simulink model "master_thesis_simulink"  (R2022a)
settings: Solver=VariableStepAuto  StartTime=0.0  StopTime=p_0p.time(end)  FixedStep=0.001  RelTol=1e-3
values from neighbouring files (symbols this model uses):
  markers_forearm = [0.00210510253906 -0.143263397217 -0.00798474121094]    [markers_forearm.mat]
  markers_shoulder = [0.010127746582 -0.151647644043 -0.0119686279297]    [markers_shoulder.mat]
undefined symbols (not defined in the file or in its folder): arm, DiscIntNeverNeededParam, Discrete, ekf, kf, LS, m, markers_hand, n, noise, q0, q0_LS, q0_model, sample_Time, selected, state_observer, Time, tSh_0_0Conf, X, Y, Z
libraries: sm_lib x2029, nesl_utility x1553, robotlib x75, ctrlSharedLib x8
(part 6 of 70)

== system master_thesis_simulink/Experiments/S1_F1_H2/Human arm1/RightHand ==
  B_wrist__setting : sm_lib/Frames and Transforms/Rigid Transform  TranslationMethod=Cartesian  TranslationStandardOffset=0  TranslationLengthUnit=m  TranslationStandardAxis=+Z  TranslationCartesianOffset=[0, arm.hand.dimensions(2)/2, 0]  TranslationROffset=0  TranslationROffsetUnits=m  TranslationZOffset=0  TranslationZOffsetUnits=m  TranslationThetaOffset=0  TranslationThetaOffsetUnits=deg  RotationMethod=None  RotationAngleUnits=deg  RotationStandardAxis=+Z  RotationAngle=0.0  RotationArbitraryAxis=[0 0 1]  FollAlignAxisA=+X  BaseAlignAxisA=+Y  FollAlignAxisB=+Y  BaseAlignAxisB=+Z  RotationSequenceAxes=BaseAxes  RotationSequence=XYZ  RotationSequenceAngles=[0, 0, 0]  RotationSequenceAnglesUnits=rad  RotationMatrix=[1 0 0; 0 1 0; 0 0 1]
  Hand : sm_lib/Body Elements/Brick Solid  GraphicAmbientColor=[0.15 0.15 0.15 1.0]  BasedOnType=Density  BrickDimensions=arm.hand.dimensions  BrickDimensionUnits=m  CenterOfMass=[0, 0, 0]  CenterOfMassUnits=m  GraphicDiffuseColor=[1.0 0.6 0.4]  Density=1000  DensityUnits=kg/m^3  DoExposeReferenceFrame=on  GraphicEmissiveColor=[0.0 0.0 0.0 1.0]  ExportEntireGeometry=off  SerializedFrames=<Frames/>  MarkerShape=Sphere  MarkerSize=10  GraphicType=FromGeometry  InertiaType=CalculateFromGeometry  Mass=0  MassUnits=kg  MomentsOfInertia=[0, 0, 0]  MomentsOfInertiaUnits=kg*m^2  GraphicOpacity=1  ProductsOfInertia=[0, 0, 0]  ProductsOfInertiaUnits=kg*m^2  GraphicShininess=75  GraphicSpecularColor=[0.5 0.5 0.5 1.0]  GraphicVisPropType=SimpleVisualProperties
  Inertia : sm_lib/Body Elements/Inertia  InertiaType=Custom  Mass=arm.hand.mass  MassUnits=kg  CenterOfMass=[0, 0, 0]  CenterOfMassUnits=m  MomentsOfInertia=arm.hand.moment_inertia  MomentsOfInertiaUnits=kg*m^2  ProductsOfInertia=[0, 0, 0]  ProductsOfInertiaUnits=kg*m^2  GraphicType=None  MarkerShape=Inertia  MarkerSize=20  GraphicVisPropType=SimpleVisualProperties  GraphicDiffuseColor=[0.5 0.5 0.5]  GraphicSpecularColor=[0.5 0.5 0.5 1.0]  GraphicAmbientColor=[0.15 0.15 0.15 1.0]  GraphicEmissiveColor=[0.0 0.0 0.0 1.0]  GraphicShininess=75  GraphicOpacity=1.0
  Mux : Mux  Inputs=3
  PS-Simulink Converter : nesl_utility/PS-Simulink Converter  PhysicalDomain=network_engine_domain  SubClassName=ps_output  LeftPortType=input  RightPortType=output  PseudoPeriodic=off  Frequencies=[]  VectorFormat=inherit  Unit=inherit  AffineConversion=off
      settings: SourceProductBaseCode=SS,PW,VE
  PS-Simulink Converter1 : nesl_utility/PS-Simulink Converter  PhysicalDomain=network_engine_domain  SubClassName=ps_output  LeftPortType=input  RightPortType=output  PseudoPeriodic=off  Frequencies=[]  VectorFormat=inherit  Unit=inherit  AffineConversion=off
      settings: SourceProductBaseCode=SS,PW,VE
  PS-Simulink Converter2 : nesl_utility/PS-Simulink Converter  PhysicalDomain=network_engine_domain  SubClassName=ps_output  LeftPortType=input  RightPortType=output  PseudoPeriodic=off  Frequencies=[]  VectorFormat=inherit  Unit=inherit  AffineConversion=off
      settings: SourceProductBaseCode=SS,PW,VE
  Reference Frame : sm_lib/Frames and Transforms/Reference Frame
  Scope : Scope
  Transform Sensor : sm_lib/Frames and Transforms/Transform Sensor  MeasurementFrame=World  SenseAngle=off  SenseAxis=off  SenseAngle1=off  SenseAngle2=off  SenseAngle3=off  SenseQ=off  SenseR=off  SenseOmegaX=off  SenseOmegaY=off  SenseOmegaZ=off  SenseOmega1=off  SenseOmega2=off  SenseOmega3=off  SenseQDot=off  SenseRDot=off  SenseAlphaX=off  SenseAlphaY=off  SenseAlphaZ=off  SenseAlpha1=off  SenseAlpha2=off  SenseAlpha3=off  SenseQDDot=off  SenseRDDot=off  SenseX=on  SenseY=on  SenseZ=on  SenseRad=off  SenseAzim=off  SenseDist=off  SenseInc=off  SenseXDot=off  SenseYDot=off  SenseZDot=off  SenseRadDot=off  SenseAzimDot=off  SenseDistDot=off  SenseIncDot=off  SenseXDDot=off  SenseYDDot=off  SenseZDDot=off  SenseRadDDot=off  SenseAzimDDot=off  SenseDistDDot=off  SenseIncDDot=off
  B_wrist : PMIOPort  Side=Left
  W : PMIOPort  Port=2  Side=Left
  wires:
  Mux/1 -> Scope/1
  PS-Simulink Converter/1 -> Mux/1  "wrist_posx"
  PS-Simulink Converter1/1 -> Mux/2  "wrist_posy"
  PS-Simulink Converter2/1 -> Mux/3  "wrist_posz"
  connections:
  B_wrist__setting/RConn1 -- Transform Sensor/RConn1 -- B_wrist/RConn1
  PS-Simulink Converter2/LConn1 -- Transform Sensor/RConn4
  PS-Simulink Converter/LConn1 -- Transform Sensor/RConn2
  PS-Simulink Converter1/LConn1 -- Transform Sensor/RConn3
  Transform Sensor/LConn1 -- W/RConn1
  B_wrist__setting/LConn1 -- Inertia/RConn1 -- Reference Frame/RConn1 -- Hand/RConn1

== system master_thesis_simulink/Experiments/S1_F1_H2/Human arm1/RightShoulder ==
  B_shoulder__F_shoulder : sm_lib/Frames and Transforms/Rigid Transform  TranslationMethod=Cartesian  TranslationStandardOffset=0  TranslationLengthUnit=m  TranslationStandardAxis=+Z  TranslationCartesianOffset=[0 -arm.shoulder.length 0]  TranslationROffset=0  TranslationROffsetUnits=m  TranslationZOffset=0  TranslationZOffsetUnits=m  TranslationThetaOffset=0  TranslationThetaOffsetUnits=deg  RotationMethod=None  RotationAngleUnits=deg  RotationStandardAxis=+Z  RotationAngle=0.0  RotationArbitraryAxis=[0 0 1]  FollAlignAxisA=+X  BaseAlignAxisA=+Y  FollAlignAxisB=+Y  BaseAlignAxisB=+Z  RotationSequenceAxes=FollowerAxes  RotationSequence=XYX  RotationSequenceAngles=[0 0 0]  RotationSequenceAnglesUnits=deg  RotationMatrix=[1 0 0; 0 1 0; 0 0 1]
  Inertia : sm_lib/Body Elements/Inertia  InertiaType=Custom  Mass=arm.shoulder.mass  MassUnits=kg  CenterOfMass=[0 0 0]  CenterOfMassUnits=m  MomentsOfInertia=arm.shoulder.moment_inertia  MomentsOfInertiaUnits=kg*m^2  ProductsOfInertia=[0 0 0]  ProductsOfInertiaUnits=kg*m^2  GraphicType=None  MarkerShape=Inertia  MarkerSize=20  GraphicVisPropType=SimpleVisualProperties  GraphicDiffuseColor=[0.5 0.5 0.5]  GraphicSpecularColor=[0.5 0.5 0.5 1.0]  GraphicAmbientColor=[0.15 0.15 0.15 1.0]  GraphicEmissiveColor=[0.0 0.0 0.0 1.0]  GraphicShininess=75  GraphicOpacity=1.0
  Mux : Mux  Inputs=3
  PS-Simulink Converter : nesl_utility/PS-Simulink Converter  PhysicalDomain=network_engine_domain  SubClassName=ps_output  LeftPortType=input  RightPortType=output  PseudoPeriodic=off  Frequencies=[]  VectorFormat=inherit  Unit=inherit  AffineConversion=off
      settings: SourceProductBaseCode=SS,PW,VE
  PS-Simulink Converter1 : nesl_utility/PS-Simulink Converter  PhysicalDomain=network_engine_domain  SubClassName=ps_output  LeftPortType=input  RightPortType=output  PseudoPeriodic=off  Frequencies=[]  VectorFormat=inherit  Unit=inherit  AffineConversion=off
      settings: SourceProductBaseCode=SS,PW,VE
  PS-Simulink Converter2 : nesl_utility/PS-Simulink Converter  PhysicalDomain=network_engine_domain  SubClassName=ps_output  LeftPortType=input  RightPortType=output  PseudoPeriodic=off  Frequencies=[]  VectorFormat=inherit  Unit=inherit  AffineConversion=off
      settings: SourceProductBaseCode=SS,PW,VE
  Reference Frame : sm_lib/Frames and Transforms/Reference Frame
  RightShoulder_rot : sm_lib/Frames and Transforms/Rigid Transform  TranslationMethod=None  TranslationStandardOffset=0  TranslationLengthUnit=m  TranslationStandardAxis=+Z  TranslationCartesianOffset=[0 0 0]  TranslationROffset=0  TranslationROffsetUnits=m  TranslationZOffset=0  TranslationZOffsetUnits=m  TranslationThetaOffset=0  TranslationThetaOffsetUnits=deg  RotationMethod=ArbitraryAxis  RotationAngleUnits=rad  RotationStandardAxis=+Z  RotationAngle=pi/2  RotationArbitraryAxis=[1 0 0]  FollAlignAxisA=+X  BaseAlignAxisA=+Y  FollAlignAxisB=+Y  BaseAlignAxisB=+Z  RotationSequenceAxes=BaseAxes  RotationSequence=XYZ  RotationSequenceAngles=[pi/2, 0, 0]  RotationSequenceAnglesUnits=rad  RotationMatrix=[1 0 0; 0 1 0; 0 0 1]
  Shoulder : sm_lib/Body Elements/Cylindrical Solid  GraphicAmbientColor=[0.15 0.15 0.15 1.0]  BasedOnType=Density  CenterOfMass=[0, 0, 0]  CenterOfMassUnits=m  GraphicDiffuseColor=[1.0 0.6 0.4]  CylinderLength=arm.shoulder.length  CylinderLengthUnits=m  CylinderRadius=arm.shoulder.radius  CylinderRadiusUnits=m  Density=1000  DensityUnits=kg/m^3  DoExposeReferenceFrame=on  GraphicEmissiveColor=[0.0 0.0 0.0 1.0]  ExportEntireGeometry=off  SerializedFrames=<Frames/>  MarkerShape=Sphere  MarkerSize=10  GraphicType=FromGeometry  InertiaType=CalculateFromGeometry  Mass=0  MassUnits=kg  MomentsOfInertia=[0, 0, 0]  MomentsOfInertiaUnits=kg*m^2  GraphicOpacity=1  ProductsOfInertia=[0, 0, 0]  ProductsOfInertiaUnits=kg*m^2  GraphicShininess=75  GraphicSpecularColor=[0.5 0.5 0.5 1.0]  GraphicVisPropType=SimpleVisualProperties
  Transform Sensor : sm_lib/Frames and Transforms/Transform Sensor  MeasurementFrame=World  SenseAngle=off  SenseAxis=off  SenseAngle1=off  SenseAngle2=off  SenseAngle3=off  SenseQ=off  SenseR=off  SenseOmegaX=off  SenseOmegaY=off  SenseOmegaZ=off  SenseOmega1=off  SenseOmega2=off  SenseOmega3=off  SenseQDot=off  SenseRDot=off  SenseAlphaX=off  SenseAlphaY=off  SenseAlphaZ=off  SenseAlpha1=off  SenseAlpha2=off  SenseAlpha3=off  SenseQDDot=off  SenseRDDot=off  SenseX=on  SenseY=on  SenseZ=on  SenseRad=off  SenseAzim=off  SenseDist=off  SenseInc=off  SenseXDot=off  SenseYDot=off  SenseZDot=off  SenseRadDot=off  SenseAzimDot=off  SenseDistDot=off  SenseIncDot=off  SenseXDDot=off  SenseYDDot=off  SenseZDDot=off  SenseRadDDot=off  SenseAzimDDot=off  SenseDistDDot=off  SenseIncDDot=off
  W_setting : sm_lib/Frames and Transforms/Rigid Transform  TranslationMethod=Cartesian  TranslationStandardOffset=0  TranslationLengthUnit=m  TranslationStandardAxis=+Z  TranslationCartesianOffset=[0 arm.shoulder.length/2 0]  TranslationROffset=0  TranslationROffsetUnits=m  TranslationZOffset=0  TranslationZOffsetUnits=m  TranslationThetaOffset=0  TranslationThetaOffsetUnits=deg  RotationMethod=None  RotationAngleUnits=rad  RotationStandardAxis=+Z  RotationAngle=pi/2  RotationArbitraryAxis=[1 0 0]  FollAlignAxisA=+X  BaseAlignAxisA=+Y  FollAlignAxisB=+Y  BaseAlignAxisB=+Z  RotationSequenceAxes=BaseAxes  RotationSequence=XYZ  RotationSequenceAngles=[pi/2, 0, 0]  RotationSequenceAnglesUnits=rad  RotationMatrix=[1 0 0; 0 1 0; 0 0 1]
  B_shoulder : PMIOPort  Side=Left
  F_shoulder : PMIOPort  Port=2  Side=Right
  W : PMIOPort  Port=3  Side=Left
  wires:
  PS-Simulink Converter/1 -> Mux/1  "shoulder_posx"
  PS-Simulink Converter1/1 -> Mux/2  "shoulder_posy"
  PS-Simulink Converter2/1 -> Mux/3  "shoulder_posz"
  connections:
  W_setting/RConn1 -- B_shoulder/RConn1 -- Transform Sensor/RConn1 -- B_shoulder__F_shoulder/LConn1
  F_shoulder/RConn1 -- B_shoulder__F_shoulder/RConn1
  PS-Simulink Converter2/LConn1 -- Transform Sensor/RConn4
  Transform Sensor/RConn2 -- PS-Simulink Converter/LConn1
  PS-Simulink Converter1/LConn1 -- Transform Sensor/RConn3
  RightShoulder_rot/LConn1 -- Shoulder/RConn1
  Transform Sensor/LConn1 -- W/RConn1
  W_setting/LConn1 -- Reference Frame/RConn1 -- Inertia/RConn1 -- RightShoulder_rot/RConn1

== system master_thesis_simulink/Experiments/S1_F1_H2/Human arm1/RightShoulder_joint ==
  note: Rotation around x
  note: Rotation around y
  note: Rotation around z
  Input : Inport
  Demux : Demux  Outputs=3
  M0 Hat : Subsystem  Commented=on
  Sx_Sy : Subsystem
  Sy_Sz : Subsystem
  W_Sx : Subsystem
  c1 : nesl_utility/Simulink-PS Converter  PhysicalDomain=network_engine_domain  SubClassName=ps_input  LeftPortType=input  RightPortType=output  PseudoPeriodic=off  Frequencies=[]  NoiseDistribution=none  NoiseParameters=[]  Unit=1  AffineConversion=off  FilteringAndDerivatives=filter  SimscapeFilterOrder=2  InputFilterTimeConstant=0.001  UdotUserProvided=0
      settings: SourceProductBaseCode=SS,PW,VE
  c2 : nesl_utility/Simulink-PS Converter  PhysicalDomain=network_engine_domain  SubClassName=ps_input  LeftPortType=input  RightPortType=output  PseudoPeriodic=off  Frequencies=[]  NoiseDistribution=none  NoiseParameters=[]  Unit=1  AffineConversion=off  FilteringAndDerivatives=filter  SimscapeFilterOrder=2  InputFilterTimeConstant=0.001  UdotUserProvided=0
      settings: SourceProductBaseCode=SS,PW,VE
  c3 : nesl_utility/Simulink-PS Converter  PhysicalDomain=network_engine_domain  SubClassName=ps_input  LeftPortType=input  RightPortType=output  PseudoPeriodic=off  Frequencies=[]  NoiseDistribution=none  NoiseParameters=[]  Unit=1  AffineConversion=off  FilteringAndDerivatives=filter  SimscapeFilterOrder=2  InputFilterTimeConstant=0.001  UdotUserProvided=0
      settings: SourceProductBaseCode=SS,PW,VE
  jRightShoulder_rotx : sm_lib/Joints/Revolute Joint  JointMode=Normal  SenseConstraintForce=off  SenseConstraintForceX=off  SenseConstraintForceY=off  SenseConstraintForceZ=off  SenseConstraintTorque=off  SenseConstraintTorqueX=off  SenseConstraintTorqueY=off  SenseConstraintTorqueZ=off  SenseTotalForce=off  SenseTotalForceX=off  SenseTotalForceY=off  SenseTotalForceZ=off  SenseTotalTorque=off  SenseTotalTorqueX=off  SenseTotalTorqueY=off  SenseTotalTorqueZ=off  CompositeWrenchDir=FollowerOnBase  CompositeWrenchFrame=BaseFrame  EquilibriumPosition=0  EquilibriumPositionUnits=deg  SpringStiffness=0  SpringStiffnessUnits=N*m/deg  DampingCoefficient=0  DampingCoefficientUnits=kg*m^2/(rad*s)  TorqueActuationMode=ComputedTorque  MotionActuationMode=InputMotion  SensePosition=on  SenseVelocity=on  SenseAcceleration=off  SenseTorqueForce=off  SenseLowerLimitTorqueForce=off  SenseUpperLimitTorqueForce=off  LowerLimitSpecify=on  LowerLimitBound=-pi/2  LowerLimitBoundUnits=rad  LowerLimitStiffness=1e4  LowerLimitStiffnessUnits=N*m/deg  LowerLimitDamping=10  LowerLimitDampingUnits=N*m/(deg/s)  LowerLimitTransitionRegionWidth=0.1  LowerLimitTransitionRegionWidthUnits=deg  UpperLimitSpecify=on  UpperLimitBound=5/9*pi  UpperLimitBoundUnits=rad  UpperLimitStiffness=1e4  UpperLimitStiffnessUnits=N*m/deg  UpperLimitDamping=10  UpperLimitDampingUnits=N*m/(deg/s)  UpperLimitTransitionRegionWidth=0.1  UpperLimitTransitionRegionWidthUnits=deg  PositionTargetSpecify=off  PositionTargetPriority=Low  PositionTargetValue=0  PositionTargetValueUnits=rad  VelocityTargetSpecify=off  VelocityTargetPriority=High  VelocityTargetValue=0  VelocityTargetValueUnits=deg/s
  jRightShoulder_roty : sm_lib/Joints/Revolute Joint  JointMode=Normal  SenseConstraintForce=off  SenseConstraintForceX=off  SenseConstraintForceY=off  SenseConstraintForceZ=off  SenseConstraintTorque=off  SenseConstraintTorqueX=off  SenseConstraintTorqueY=off  SenseConstraintTorqueZ=off  SenseTotalForce=off  SenseTotalForceX=off  SenseTotalForceY=off  SenseTotalForceZ=off  SenseTotalTorque=off  SenseTotalTorqueX=off  SenseTotalTorqueY=off  SenseTotalTorqueZ=off  CompositeWrenchDir=FollowerOnBase  CompositeWrenchFrame=BaseFrame  EquilibriumPosition=0  EquilibriumPositionUnits=deg  SpringStiffness=0  SpringStiffnessUnits=N*m/deg  DampingCoefficient=0  DampingCoefficientUnits=kg*m^2/(rad*s)  TorqueActuationMode=ComputedTorque  MotionActuationMode=InputMotion  SensePosition=on  SenseVelocity=on  SenseAcceleration=off  SenseTorqueForce=off  SenseLowerLimitTorqueForce=off  SenseUpperLimitTorqueForce=off  LowerLimitSpecify=on  LowerLimitBound=-pi/10  LowerLimitBoundUnits=rad  LowerLimitStiffness=1e4  LowerLimitStiffnessUnits=N*m/deg  LowerLimitDamping=10  LowerLimitDampingUnits=N*m/(deg/s)  LowerLimitTransitionRegionWidth=0.1  LowerLimitTransitionRegionWidthUnits=deg  UpperLimitSpecify=on  UpperLimitBound=pi/10  UpperLimitBoundUnits=rad  UpperLimitStiffness=1e4  UpperLimitStiffnessUnits=N*m/deg  UpperLimitDamping=10  UpperLimitDampingUnits=N*m/(deg/s)  UpperLimitTransitionRegionWidth=0.1  UpperLimitTransitionRegionWidthUnits=deg  PositionTargetSpecify=off  PositionTargetPriority=Low  PositionTargetValue=0  PositionTargetValueUnits=rad  VelocityTargetSpecify=off  VelocityTargetPriority=High  VelocityTargetValue=0  VelocityTargetValueUnits=deg/s
  jRightShoulder_rotz : sm_lib/Joints/Revolute Joint  JointMode=Normal  SenseConstraintForce=off  SenseConstraintForceX=off  SenseConstraintForceY=off  SenseConstraintForceZ=off  SenseConstraintTorque=off  SenseConstraintTorqueX=off  SenseConstraintTorqueY=off  SenseConstraintTorqueZ=off  SenseTotalForce=off  SenseTotalForceX=off  SenseTotalForceY=off  SenseTotalForceZ=off  SenseTotalTorque=off  SenseTotalTorqueX=off  SenseTotalTorqueY=off  SenseTotalTorqueZ=off  CompositeWrenchDir=FollowerOnBase  CompositeWrenchFrame=BaseFrame  EquilibriumPosition=0  EquilibriumPositionUnits=deg  SpringStiffness=0  SpringStiffnessUnits=N*m/deg  DampingCoefficient=0.1  DampingCoefficientUnits=kg*m^2/(rad*s)  TorqueActuationMode=ComputedTorque  MotionActuationMode=InputMotion  SensePosition=on  SenseVelocity=on  SenseAcceleration=off  SenseTorqueForce=off  SenseLowerLimitTorqueForce=off  SenseUpperLimitTorqueForce=off  LowerLimitSpecify=on  LowerLimitBound=-pi/10  LowerLimitBoundUnits=rad  LowerLimitStiffness=1e4  LowerLimitStiffnessUnits=N*m/deg  LowerLimitDamping=10  LowerLimitDampingUnits=N*m/(deg/s)  LowerLimitTransitionRegionWidth=0.1  LowerLimitTransitionRegionWidthUnits=deg  UpperLimitSpecify=on  UpperLimitBound=pi/10  UpperLimitBoundUnits=rad  UpperLimitStiffness=1e4  UpperLimitStiffnessUnits=N*m/deg  UpperLimitDamping=10  UpperLimitDampingUnits=N*m/(deg/s)  UpperLimitTransitionRegionWidth=0.1  UpperLimitTransitionRegionWidthUnits=deg  PositionTargetSpecify=off  PositionTargetPriority=Low  PositionTargetValue=0  PositionTargetValueUnits=rad  VelocityTargetSpecify=off  VelocityTargetPriority=High  VelocityTargetValue=0  VelocityTargetValueUnits=deg/s
  B_shoulder : PMIOPort  Side=Right
  W : PMIOPort  Port=2  Side=Left
  wires:
  Input/1 -> Demux/1
  Demux/1 -> c1/1
  Demux/2 -> c2/1
  Demux/3 -> c3/1
  connections:
  jRightShoulder_rotx/RConn1 -- Sx_Sy/LConn1
  B_shoulder/RConn1 -- jRightShoulder_rotz/RConn1
  Sy_Sz/RConn1 -- jRightShoulder_rotz/LConn1
  W_Sx/RConn1 -- jRightShoulder_rotx/LConn1
  Sx_Sy/RConn1 -- jRightShoulder_roty/LConn1
  Sy_Sz/LConn1 -- jRightShoulder_roty/RConn1
  ?
  ?
  ?
  W/RConn1 -- M0 Hat/LConn1 -- M0 Hat/RConn1 -- W_Sx/LConn1
  c1/RConn1 -- jRightShoulder_rotx/LConn2
  c2/RConn1 -- jRightShoulder_roty/LConn2
  c3/RConn1 -- jRightShoulder_rotz/LConn2

== system master_thesis_simulink/Experiments/S1_F1_H2/Human arm1/Wrist_joint ==
  Input : Inport
  Demux : Demux  Outputs=3
  F_elbow__Wx : Subsystem
  Wx_Wy : Subsystem
  Wy_Wz : Subsystem
  c1 : nesl_utility/Simulink-PS Converter  PhysicalDomain=network_engine_domain  SubClassName=ps_input  LeftPortType=input  RightPortType=output  PseudoPeriodic=off  Frequencies=[]  NoiseDistribution=none  NoiseParameters=[]  Unit=1  AffineConversion=off  FilteringAndDerivatives=filter  SimscapeFilterOrder=2  InputFilterTimeConstant=0.001  UdotUserProvided=0
      settings: SourceProductBaseCode=SS,PW,VE
  c2 : nesl_utility/Simulink-PS Converter  PhysicalDomain=network_engine_domain  SubClassName=ps_input  LeftPortType=input  RightPortType=output  PseudoPeriodic=off  Frequencies=[]  NoiseDistribution=none  NoiseParameters=[]  Unit=1  AffineConversion=off  FilteringAndDerivatives=filter  SimscapeFilterOrder=2  InputFilterTimeConstant=0.001  UdotUserProvided=0
      settings: SourceProductBaseCode=SS,PW,VE
  c3 : nesl_utility/Simulink-PS Converter  PhysicalDomain=network_engine_domain  SubClassName=ps_input  LeftPortType=input  RightPortType=output  PseudoPeriodic=off  Frequencies=[]  NoiseDistribution=none  NoiseParameters=[]  Unit=1  AffineConversion=off  FilteringAndDerivatives=filter  SimscapeFilterOrder=2  InputFilterTimeConstant=0.001  UdotUserProvided=0
      settings: SourceProductBaseCode=SS,PW,VE
  jRightWrist_rotx : sm_lib/Joints/Revolute Joint  JointMode=Normal  SenseConstraintForce=off  SenseConstraintForceX=off  SenseConstraintForceY=off  SenseConstraintForceZ=off  SenseConstraintTorque=off  SenseConstraintTorqueX=off  SenseConstraintTorqueY=off  SenseConstraintTorqueZ=off  SenseTotalForce=off  SenseTotalForceX=off  SenseTotalForceY=off  SenseTotalForceZ=off  SenseTotalTorque=off  SenseTotalTorqueX=off  SenseTotalTorqueY=off  SenseTotalTorqueZ=off  CompositeWrenchDir=FollowerOnBase  CompositeWrenchFrame=BaseFrame  EquilibriumPosition=0  EquilibriumPositionUnits=deg  SpringStiffness=0  SpringStiffnessUnits=N*m/deg  DampingCoefficient=0.01  DampingCoefficientUnits=kg*m^2/(rad*s)  TorqueActuationMode=ComputedTorque  MotionActuationMode=InputMotion  SensePosition=on  SenseVelocity=on  SenseAcceleration=off  SenseTorqueForce=off  SenseLowerLimitTorqueForce=off  SenseUpperLimitTorqueForce=off  LowerLimitSpecify=on  LowerLimitBound=-pi/4  LowerLimitBoundUnits=rad  LowerLimitStiffness=1e4  LowerLimitStiffnessUnits=N*m/deg  LowerLimitDamping=10  LowerLimitDampingUnits=N*m/(deg/s)  LowerLimitTransitionRegionWidth=0.1  LowerLimitTransitionRegionWidthUnits=deg  UpperLimitSpecify=on  UpperLimitBound=pi/3  UpperLimitBoundUnits=rad  UpperLimitStiffness=1e4  UpperLimitStiffnessUnits=N*m/deg  UpperLimitDamping=10  UpperLimitDampingUnits=N*m/(deg/s)  UpperLimitTransitionRegionWidth=0.1  UpperLimitTransitionRegionWidthUnits=deg  PositionTargetSpecify=off  PositionTargetPriority=Low  PositionTargetValue=0  PositionTargetValueUnits=rad  VelocityTargetSpecify=off  VelocityTargetPriority=High  VelocityTargetValue=0  VelocityTargetValueUnits=deg/s
  jRightWrist_roty : sm_lib/Joints/Revolute Joint  JointMode=Normal  SenseConstraintForce=off  SenseConstraintForceX=off  SenseConstraintForceY=off  SenseConstraintForceZ=off  SenseConstraintTorque=off  SenseConstraintTorqueX=off  SenseConstraintTorqueY=off  SenseConstraintTorqueZ=off  SenseTotalForce=off  SenseTotalForceX=off  SenseTotalForceY=off  SenseTotalForceZ=off  SenseTotalTorque=off  SenseTotalTorqueX=off  SenseTotalTorqueY=off  SenseTotalTorqueZ=off  CompositeWrenchDir=FollowerOnBase  CompositeWrenchFrame=BaseFrame  EquilibriumPosition=0  EquilibriumPositionUnits=deg  SpringStiffness=0  SpringStiffnessUnits=N*m/deg  DampingCoefficient=0  DampingCoefficientUnits=kg*m^2/(rad*s)  TorqueActuationMode=ComputedTorque  MotionActuationMode=InputMotion  SensePosition=on  SenseVelocity=on  SenseAcceleration=off  SenseTorqueForce=off  SenseLowerLimitTorqueForce=off  SenseUpperLimitTorqueForce=off  LowerLimitSpecify=on  LowerLimitBound=-pi/10  LowerLimitBoundUnits=rad  LowerLimitStiffness=1e4  LowerLimitStiffnessUnits=N*m/deg  LowerLimitDamping=10  LowerLimitDampingUnits=N*m/(deg/s)  LowerLimitTransitionRegionWidth=0.1  LowerLimitTransitionRegionWidthUnits=deg  UpperLimitSpecify=on  UpperLimitBound=pi/10  UpperLimitBoundUnits=rad  UpperLimitStiffness=1e4  UpperLimitStiffnessUnits=N*m/deg  UpperLimitDamping=10  UpperLimitDampingUnits=N*m/(deg/s)  UpperLimitTransitionRegionWidth=0.1  UpperLimitTransitionRegionWidthUnits=deg  PositionTargetSpecify=off  PositionTargetPriority=Low  PositionTargetValue=0  PositionTargetValueUnits=rad  VelocityTargetSpecify=off  VelocityTargetPriority=High  VelocityTargetValue=0  VelocityTargetValueUnits=deg/s
  jRightWrist_rotz : sm_lib/Joints/Revolute Joint  JointMode=Normal  SenseConstraintForce=off  SenseConstraintForceX=off  SenseConstraintForceY=off  SenseConstraintForceZ=off  SenseConstraintTorque=off  SenseConstraintTorqueX=off  SenseConstraintTorqueY=off  SenseConstraintTorqueZ=off  SenseTotalForce=off  SenseTotalForceX=off  SenseTotalForceY=off  SenseTotalForceZ=off  SenseTotalTorque=off  SenseTotalTorqueX=off  SenseTotalTorqueY=off  SenseTotalTorqueZ=off  CompositeWrenchDir=FollowerOnBase  CompositeWrenchFrame=BaseFrame  EquilibriumPosition=0  EquilibriumPositionUnits=deg  SpringStiffness=0  SpringStiffnessUnits=N*m/deg  DampingCoefficient=0  DampingCoefficientUnits=kg*m^2/(rad*s)  TorqueActuationMode=ComputedTorque  MotionActuationMode=InputMotion  SensePosition=on  SenseVelocity=on  SenseAcceleration=off  SenseTorqueForce=off  SenseLowerLimitTorqueForce=off  SenseUpperLimitTorqueForce=off  LowerLimitSpecify=on  LowerLimitBound=-20  LowerLimitBoundUnits=deg  LowerLimitStiffness=1e4  LowerLimitStiffnessUnits=N*m/deg  LowerLimitDamping=10  LowerLimitDampingUnits=N*m/(deg/s)  LowerLimitTransitionRegionWidth=0.1  LowerLimitTransitionRegionWidthUnits=deg  UpperLimitSpecify=on  UpperLimitBound=pi/6  UpperLimitBoundUnits=rad  UpperLimitStiffness=1e4  UpperLimitStiffnessUnits=N*m/deg  UpperLimitDamping=10  UpperLimitDampingUnits=N*m/(deg/s)  UpperLimitTransitionRegionWidth=0.1  UpperLimitTransitionRegionWidthUnits=deg  PositionTargetSpecify=off  PositionTargetPriority=Low  PositionTargetValue=0  PositionTargetValueUnits=rad  VelocityTargetSpecify=off  VelocityTargetPriority=High  VelocityTargetValue=0  VelocityTargetValueUnits=deg/s
  B_wrist : PMIOPort  Side=Right
  F_elbow : PMIOPort  Port=2  Side=Left
  wires:
  Demux/1 -> c1/1
  Input/1 -> Demux/1
  Demux/2 -> c2/1
  Demux/3 -> c3/1
  connections:
  F_elbow__Wx/RConn1 -- jRightWrist_rotx/LConn1
  jRightWrist_rotx/RConn1 -- Wx_Wy/LConn1
  Wy_Wz/RConn1 -- jRightWrist_rotz/LConn1
  jRightWrist_roty/LConn1 -- Wx_Wy/RConn1
  jRightWrist_roty/RConn1 -- Wy_Wz/LConn1
  F_elbow__Wx/LConn1 -- F_elbow/RConn1
  B_wrist/RConn1 -- jRightWrist_rotz/RConn1
  ?
  ?
  ?
  c1/RConn1 -- jRightWrist_rotx/LConn2
  c2/RConn1 -- jRightWrist_roty/LConn2
  c3/RConn1 -- jRightWrist_rotz/LConn2

== system master_thesis_simulink/Experiments/S1_F1_H2/Model validation/Display ==
  p_0' : Inport
  p_FK : Inport  Port=2
  Demux : Demux
  Demux1 : Demux
  Mux{,1..3} (4 alike) : Mux  Inputs=2
  Mux8 : Mux
  Scope{,1..3} (4 alike) : Scope
  To Workspace : ToWorkspace  VariableName=p0p_vs_pFK  SaveFormat=Structure With Time  SampleTime=-1
  wires:
  p_0'/1 -> Demux/1
  p_FK/1 -> Demux1/1
  Demux/1 -> Mux/1  "M1_0"
  Demux1/1 -> Mux/2  "M1_FK"
  Mux/1 -> Mux8/1, Scope/1
  Demux/2 -> Mux1/1  "M2_0"
  Demux1/2 -> Mux1/2  "M2_FK"
  Demux/3 -> Mux2/1  "M3_0"
  Demux1/3 -> Mux2/2  "M3_FK"
  Mux2/1 -> Mux8/3, Scope1/1
  Demux/4 -> Mux3/1  "M4_0"
  Demux1/4 -> Mux3/2  "M4_FK"
  Mux1/1 -> Mux8/2, Scope2/1
  Mux3/1 -> Scope3/1, Mux8/4
  Mux8/1 -> To Workspace/1

== system master_thesis_simulink/Experiments/S1_F1_H2/Model validation/Human arm ==
  note: B_shoulder
  note: ELBOW-FOREARM
  note: SHOULDER
  note: WRIST-HAND
  Elbow_joint : Subsystem
  Markers : Subsystem  Commented=on
  Mechanism Configuration : sm_lib/Utilities/Mechanism Configuration  UniformGravity=Constant  GravityVector=[0 0 -9.80665]  GravityUnits=m/s^2  LinearizationDelta=0.001  JointModeTransitionNonlinearIterations=2
  Mux : Mux  Inputs=m
  Mux1 : Mux  Inputs=m
  RightForeArm : Subsystem
  RightHand : Subsystem
  RightShoulder : Subsystem
  RightShoulder_joint : Subsystem
  Solver Configuration1 : nesl_utility/Solver Configuration  PhysicalDomain=network_engine_domain  SubClassName=solver  LeftPortType=input  RightPortType=generic  Tones=[]  Harmonics=[]  SimulateNoise=off  Profile=off  UseLocalSampling=off  EnableSwitchedLinearOptims=on  FrequencyDomain=off  UseCCode=off  RelTol=0.001  AbsTol=0.001  MinStep=1e-09  ToWorkspace=off  RevertToSquareIcSolve=off  NumHomotopyIterations=100  PhasorMode=off  PhasorModeNumHarmonics=1  IndexReductionMethod=DerivativeReplacement  DoDC=off  ResidualTolerance=1e-09  UseLocalSolver=on  LocalSolverChoice=NE_BACKWARD_EULER_ADVANCER  LocalSolverSampleTime=sample_Time  DoFixedCost=on  MaxNonlinIter=3  MaxModeIter=2  ComputeImpulses=off  ImpulseIterations=2  LinearAlgebra=auto  LinearAlgebraNumThread=0  EquationFormulation=NE_TIME_EF  DelaysMemoryBudget=1024  AutomaticFiltering=on  FilteringTimeConstant=0.001  PartitionStorageMethod=AS_NEEDED  PartitionMemoryBudget=1024  PartitionMethod=ROBUST
      settings: SourceProductBaseCode=SS,PW,VE
  World Frame : sm_lib/Frames and Transforms/World Frame
  Wrist_joint : Subsystem
  p : Outport
  pdot : Outport  Port=2
  wires:
  Mux/1 -> p/1
  Mux1/1 -> pdot/1
  [p_1] -> Mux/1
  [pdot_1] -> Mux1/1
  [p_2] -> Mux/2
  [pdot_2] -> Mux1/2
  [p_3] -> Mux/3
  [pdot_3] -> Mux1/3
  [p_4] -> Mux/4
  [pdot_4] -> Mux1/4
  connections:
  RightForeArm/LConn2 -- RightHand/LConn2 -- RightShoulder/LConn2 -- Mechanism Configuration/RConn1 -- World Frame/RConn1 -- RightShoulder_joint/LConn1 -- Solver Configuration1/RConn1
  Elbow_joint/RConn1 -- RightForeArm/LConn1
  RightHand/LConn1 -- Wrist_joint/RConn1
  Wrist_joint/LConn1 -- RightForeArm/RConn1
  RightShoulder/RConn1 -- Elbow_joint/LConn1
  RightShoulder_joint/RConn1 -- RightShoulder/LConn1

== system master_thesis_simulink/Experiments/S1_F2_H2/Experiments/EKF ==
  p_0' : Inport
  v_0' : Inport  Port=2
  markers shoulder : Inport  Port=3
  markers forearm : Inport  Port=4
  markers hand : Inport  Port=5
  Action Port : ActionPort  ActionPortLabel=case [ 2 ]:
  Extended Kalman Filter : MATLAB Function  TreatAsAtomicUnit=on
  Gain1 : Gain  Gain=180/pi
  Scope1 : Scope
  Scope2 : Scope
  Scope4 : Scope
  Terminator : Terminator
  error_FK__EKF : ToWorkspace  VariableName=error_FK__EKF  SaveFormat=Structure With Time  SampleTime=-1
  p_0p - Phi(q_EKF) : MATLAB Function  TreatAsAtomicUnit=on
  p_1 : InportShadow
  p_2 : ToWorkspace  VariableName=p_0p  SaveFormat=Structure With Time  SampleTime=-1
  q_EKF : ToWorkspace  VariableName=q_EKF  SaveFormat=Structure With Time  SampleTime=-1
  v_1 : ToWorkspace  VariableName=v_0p  SaveFormat=Structure With Time  SampleTime=-1
  wires:
  Extended Kalman Filter/2(Pk) -> Terminator/1
  [q_EKF] -> p_0p - Phi(q_EKF)/2(q_EKF)
  markers shoulder/1 -> Extended Kalman Filter/3(shoulder_variables), p_0p - Phi(q_EKF)/3(shoulder_variables)
  markers forearm/1 -> Extended Kalman Filter/4(forearm_variables), p_0p - Phi(q_EKF)/4(forearm_variables)
  markers hand/1 -> Extended Kalman Filter/5(hand_variables), p_0p - Phi(q_EKF)/5(hand_variables)
  Gain1/1 -> Scope1/1, q_EKF/1  "q_EKF [deg]"
  p_0p - Phi(q_EKF)/1(error_FK) -> Scope2/1, error_FK__EKF/1
  p_1/1 -> p_0p - Phi(q_EKF)/1(p_0p)
  Extended Kalman Filter/1(qk) -> Scope4/1, Gain1/1, [q_EKF]
  v_0'/1 -> Extended Kalman Filter/2(v_0p), v_1/1
  p_0'/1 -> p_2/1, Extended Kalman Filter/1(p_0p)

== system master_thesis_simulink/Experiments/S1_F2_H2/Experiments/Human arm ==
  note: B_shoulder
  note: ELBOW-FOREARM
  note: SHOULDER
  note: WRIST-HAND
  Elbow_joint : Subsystem
  From3 : From  Commented=on  GotoTag=pShoulder_0  TagVisibility=global
  From4 : From  Commented=on  GotoTag=pForearm_0  TagVisibility=global
  From5 : From  Commented=on  GotoTag=pHand_0  TagVisibility=global
  Goto1 : Goto  Commented=on  GotoTag=pShoulder_i_0  TagVisibility=global
  Goto2 : Goto  Commented=on  GotoTag=pForearm_i_0  TagVisibility=global
  Goto3 : Goto  Commented=on  GotoTag=pHand_i_0  TagVisibility=global
  MATLAB Function2 : MATLAB Function  Commented=on  TreatAsAtomicUnit=on
  MATLAB Function3 : MATLAB Function  Commented=on  TreatAsAtomicUnit=on
  MATLAB Function4 : MATLAB Function  Commented=on  TreatAsAtomicUnit=on
  Markers : Subsystem  Commented=on
  Mechanism Configuration : sm_lib/Utilities/Mechanism Configuration  UniformGravity=Constant  GravityVector=[0 0 -9.80665]  GravityUnits=m/s^2  LinearizationDelta=0.001  JointModeTransitionNonlinearIterations=2
  Mux : Mux  Inputs=m
  Mux1 : Mux  Inputs=m
  RightForeArm : Subsystem
  RightHand : Subsystem
  RightShoulder : Subsystem
  RightShoulder_joint : Subsystem
  Solver Configuration1 : nesl_utility/Solver Configuration  PhysicalDomain=network_engine_domain  SubClassName=solver  LeftPortType=input  RightPortType=generic  Tones=[]  Harmonics=[]  SimulateNoise=off  Profile=off  UseLocalSampling=off  EnableSwitchedLinearOptims=on  FrequencyDomain=off  UseCCode=off  RelTol=0.001  AbsTol=0.001  MinStep=1e-09  ToWorkspace=off  RevertToSquareIcSolve=off  NumHomotopyIterations=100  PhasorMode=off  PhasorModeNumHarmonics=1  IndexReductionMethod=DerivativeReplacement  DoDC=off  ResidualTolerance=1e-09  UseLocalSolver=off  LocalSolverChoice=NE_BACKWARD_EULER_ADVANCER  LocalSolverSampleTime=0.001  DoFixedCost=off  MaxNonlinIter=3  MaxModeIter=2  ComputeImpulses=off  ImpulseIterations=2  LinearAlgebra=auto  LinearAlgebraNumThread=0  EquationFormulation=NE_TIME_EF  DelaysMemoryBudget=1024  AutomaticFiltering=on  FilteringTimeConstant=0.001  PartitionStorageMethod=AS_NEEDED  PartitionMemoryBudget=1024  PartitionMethod=ROBUST
      settings: SourceProductBaseCode=SS,PW,VE
  World Frame : sm_lib/Frames and Transforms/World Frame
  Wrist_joint : Subsystem
  p : Outport
  pdot : Outport  Port=2
  wires:
  Mux/1 -> p/1
  Mux1/1 -> pdot/1
  From3/1 -> MATLAB Function2/1(shoulder)
  MATLAB Function2/1(y) -> Goto1/1
  MATLAB Function3/1(y) -> Goto2/1
  From4/1 -> MATLAB Function3/1(forearm)
  From5/1 -> MATLAB Function4/1(hand)
  MATLAB Function4/1(y) -> Goto3/1
  connections:
  Mechanism Configuration/RConn1 -- RightShoulder_joint/LConn1 -- RightForeArm/LConn2 -- RightHand/LConn2 -- RightShoulder/LConn2 -- Solver Configuration1/RConn1 -- World Frame/RConn1
  Elbow_joint/RConn1 -- RightForeArm/LConn1
  RightHand/LConn1 -- Wrist_joint/RConn1
  Wrist_joint/LConn1 -- RightForeArm/RConn1
  RightShoulder/RConn1 -- Elbow_joint/LConn1
  RightShoulder_joint/RConn1 -- RightShoulder/LConn1

== system master_thesis_simulink/Experiments/S1_F2_H2/Experiments/Human arm_exp ==
  note: B_shoulder
  note: SHOULDER
  note: ELBOW-FOREARM
  note: WRIST-HAND
  Elbow_joint : Subsystem
  Markers : Subsystem  Commented=on
  Mechanism Configuration : sm_lib/Utilities/Mechanism Configuration  UniformGravity=Constant  GravityVector=[0 0 -9.80665]  GravityUnits=m/s^2  LinearizationDelta=0.001  JointModeTransitionNonlinearIterations=2
  Mux : Mux  Inputs=m
  Mux1 : Mux  Inputs=m
  RightForeArm : Subsystem
  RightHand : Subsystem
  RightShoulder : Subsystem
  RightShoulder_joint : Subsystem
  Solver Configuration1 : nesl_utility/Solver Configuration  PhysicalDomain=network_engine_domain  SubClassName=solver  LeftPortType=input  RightPortType=generic  Tones=[]  Harmonics=[]  SimulateNoise=off  Profile=off  UseLocalSampling=off  EnableSwitchedLinearOptims=on  FrequencyDomain=off  UseCCode=off  RelTol=0.001  AbsTol=0.001  MinStep=1e-09  ToWorkspace=off  RevertToSquareIcSolve=off  NumHomotopyIterations=100  PhasorMode=off  PhasorModeNumHarmonics=1  IndexReductionMethod=DerivativeReplacement  DoDC=off  ResidualTolerance=1e-09  UseLocalSolver=off  LocalSolverChoice=NE_BACKWARD_EULER_ADVANCER  LocalSolverSampleTime=0.001  DoFixedCost=off  MaxNonlinIter=3  MaxModeIter=2  ComputeImpulses=off  ImpulseIterations=2  LinearAlgebra=auto  LinearAlgebraNumThread=0  EquationFormulation=NE_TIME_EF  DelaysMemoryBudget=1024  AutomaticFiltering=on  FilteringTimeConstant=0.001  PartitionStorageMethod=AS_NEEDED  PartitionMemoryBudget=1024  PartitionMethod=ROBUST
      settings: SourceProductBaseCode=SS,PW,VE
  World Frame : sm_lib/Frames and Transforms/World Frame
  Wrist_joint : Subsystem
  p : Outport
  pdot : Outport  Port=2
  wires:
  Mux/1 -> p/1
  Mux1/1 -> pdot/1
  connections:
  RightShoulder/LConn1 -- RightShoulder_joint/RConn1
  RightHand/LConn1 -- Wrist_joint/RConn1
  Elbow_joint/LConn1 -- RightShoulder/RConn1
  Wrist_joint/LConn1 -- RightForeArm/RConn1
  RightForeArm/LConn2 -- RightHand/LConn2 -- RightShoulder/LConn2 -- Solver Configuration1/RConn1 -- Mechanism Configuration/RConn1 -- World Frame/RConn1 -- RightShoulder_joint/LConn1
  Elbow_joint/RConn1 -- RightForeArm/LConn1

== system master_thesis_simulink/Experiments/S1_F2_H2/Experiments/KF ==
  p_0' : Inport
  v_0' : Inport  Port=2
  Action Port : ActionPort
  Discrete State-Space : DiscreteStateSpace  Commented=on  A=kf.F  B=kf.G  C=kf.H  D=kf.J  InitialCondition=q0_model - kf.q_eq  SampleTime=sample_Time
  Kalman Filter : MATLAB Function  Commented=on  TreatAsAtomicUnit=on
  Kalman Filter1 : ctrlSharedLib/Kalman Filter  TimeDomain=Discrete-Time  UseCurrentEstimator=on  ModelSource=Individual A, B, C, D matrices  ModelSourceVariable=ss(0.95,1,1,0,1)  A=kf.F  B=kf.G  C=kf.H  D=kf.J  NumberOfStates=1  NumberOfInputs=1  NumberOfOutputs=1  InitialEstimateSource=Dialog  X0=kf.Delta_q0  P0=kf.P0  UseK=off  UseGH=off  NumberOfProcessNoiseInputs=1  G=1  TimeInvariantG=on  H=0  TimeInvariantH=on  Q=noise.Q  TimeInvariantQ=on  R=noise.R  TimeInvariantR=on  N=0  TimeInvariantN=on  AddInputPort=on  AddEnablePort=off  OutputEstimatedY=off  OutputP=off  Ts=sample_Time
  MATLAB Function : MATLAB Function  Commented=on  TreatAsAtomicUnit=on
  R : RandomNumber  Commented=on  Variance=diag(noise.R)  Seed=noise.R_seed  SampleTime=sample_Time
  Scope : Scope  NumInputPorts=2
  Sum1 : Sum  Commented=on  Inputs=++|
  Sum2 : Sum  Commented=on  Inputs=++|
  Sum3 : Sum  Inputs=|+-
  Sum4 : Sum  Inputs=++|
  Sum5 : Sum  Commented=on  Inputs=|++
  Sum6 : Sum  Inputs=|+-
  Terminator1 : Terminator  Commented=on
  Terminator2 : Terminator
  Terminator3 : Terminator
  To Workspace1 : ToWorkspace  VariableName=qk_kf  SaveFormat=Structure With Time  SampleTime=-1
  p_eq : Constant  Value=kf.p_eq  SampleTime=sample_Time
  q_eq : Constant  Commented=on  Value=kf.q_eq  SampleTime=sample_Time
  q_eq1 : Constant  Value=kf.q_eq  SampleTime=sample_Time
  trial : Subsystem  Commented=on
  u_eq : Constant  Value=kf.u_eq  SampleTime=sample_Time
  q_KF : Outport
  wires:
  Sum6/1 -> Kalman Filter1/2, Kalman Filter/1(Delta_pk)  "Delta_uk"
  p_eq/1 -> Sum6/2  "u_eqk"
  p_0'/1 -> Sum6/1
  MATLAB Function/1(n_k) -> Sum5/1
  Sum4/1 -> Scope/2, To Workspace1/1, q_KF/1  "kf simulink"
  q_eq1/1 -> Sum4/1
  Kalman Filter1/1 -> Sum4/2
  trial/2(q_KF) -> Terminator3/1
  trial/1(q_OBS) -> Terminator2/1
  Sum2/1 -> Scope/1  "kf"
  Kalman Filter/2(Pk) -> Terminator1/1
  q_eq/1 -> Sum2/1
  Kalman Filter/1(Delta_qk) -> Sum2/2  "Delta qk"
  R/1 -> Sum1/1
  Discrete State-Space/1 -> Sum1/2
  Sum3/1 -> Sum5/2, trial/1(Delta uk), Kalman Filter/2(Delta_uk), Kalman Filter1/1  "Delta _uk"
  u_eq/1 -> Sum3/2  "u_eqk"
  v_0'/1 -> Sum3/1

== system master_thesis_simulink/Experiments/S1_F2_H2/Experiments/LS ==
  p_0' : Inport
  v_0' : Inport  Port=2
  markers shoulder : Inport  Port=3
  markers forearm : Inport  Port=4
  markers hand : Inport  Port=5
  Action Port : ActionPort
  Discrete-Time Integrator : DiscreteIntegrator  InitialCondition=q0_LS  SampleTime=-1  LimitOutput=on  UpperSaturationLimit=4*pi  LowerSaturationLimit=-4*pi  ICPrevOutput=DiscIntNeverNeededParam  ICPrevScaledInput=DiscIntNeverNeededParam
  Gain : Gain  Gain=180/pi
  LS : MATLAB Function  TreatAsAtomicUnit=on
  Scope1 : Scope
  Scope2 : Scope
  error_FK__LS : ToWorkspace  VariableName=error_FK__LS  SaveFormat=Structure With Time  SampleTime=-1
  p_0 - Phi(q_LS) : MATLAB Function  TreatAsAtomicUnit=on
  q_LS : ToWorkspace  VariableName=q_LS  SaveFormat=Structure With Time  SampleTime=-1
  tag scope: q_LS=global
  wires:
  v_0'/1 -> LS/2(v_0)
  [q_LS] -> p_0 - Phi(q_LS)/2(q_LS), LS/1(q)
  LS/1(qdot_LS) -> Discrete-Time Integrator/1
  markers shoulder/1 -> p_0 - Phi(q_LS)/3(shoulder_variables), LS/3(shoulder_variables)
  markers forearm/1 -> p_0 - Phi(q_LS)/4(forearm_variables), LS/4(forearm_variables)
  markers hand/1 -> p_0 - Phi(q_LS)/5(hand_variables), LS/5(hand_variables)
  Discrete-Time Integrator/1 -> Gain/1, [q_LS]  "q_LS"
  Gain/1 -> q_LS/1, Scope2/1  "q_LS [deg]"
  p_0 - Phi(q_LS)/1(error_FK) -> Scope1/1, error_FK__LS/1
  p_0'/1 -> p_0 - Phi(q_LS)/1(p_0)

== system master_thesis_simulink/Experiments/S1_F2_H2/Model validation/Display ==
  p_0' : Inport
  p_FK : Inport  Port=2
  Demux : Demux  Outputs=5
  Demux1 : Demux  Outputs=5
  Mux{,1..4} (5 alike) : Mux  Inputs=2
  Mux8 : Mux  Inputs=5
  Scope{,1..4} (5 alike) : Scope
  To Workspace : ToWorkspace  VariableName=p0p_vs_pFK  SaveFormat=Structure With Time  SampleTime=-1
  wires:
  p_0'/1 -> Demux/1
  p_FK/1 -> Demux1/1
  Demux/1 -> Mux/1  "M1_0"
  Demux1/1 -> Mux/2  "M1_FK"
  Mux/1 -> Mux8/1, Scope/1
  Demux/2 -> Mux1/1  "M2_0"
  Demux1/2 -> Mux1/2  "M2_FK"
  Demux/3 -> Mux2/1  "M3_0"
  Demux1/3 -> Mux2/2  "M3_FK"
  Mux2/1 -> Mux8/3, Scope1/1
  Demux/4 -> Mux3/1  "M4_0"
  Demux1/4 -> Mux3/2  "M4_FK"
  Mux1/1 -> Mux8/2, Scope2/1
  Mux3/1 -> Scope3/1, Mux8/4
  Mux8/1 -> To Workspace/1
  Demux/5 -> Mux4/1
  Demux1/5 -> Mux4/2
  Mux4/1 -> Mux8/5, Scope4/1

== system master_thesis_simulink/Experiments/S1_F2_H2/Model validation/Human arm ==
  note: B_shoulder
  note: ELBOW-FOREARM
  note: SHOULDER
  note: WRIST-HAND
  Elbow_joint : Subsystem
  Markers : Subsystem  Commented=on
  Mechanism Configuration : sm_lib/Utilities/Mechanism Configuration  UniformGravity=Constant  GravityVector=[0 0 -9.80665]  GravityUnits=m/s^2  LinearizationDelta=0.001  JointModeTransitionNonlinearIterations=2
  Mux : Mux  Inputs=m
  Mux1 : Mux  Inputs=m
  RightForeArm : Subsystem
  RightHand : Subsystem
  RightShoulder : Subsystem
  RightShoulder_joint : Subsystem
  Solver Configuration1 : nesl_utility/Solver Configuration  PhysicalDomain=network_engine_domain  SubClassName=solver  LeftPortType=input  RightPortType=generic  Tones=[]  Harmonics=[]  SimulateNoise=off  Profile=off  UseLocalSampling=off  EnableSwitchedLinearOptims=on  FrequencyDomain=off  UseCCode=off  RelTol=0.001  AbsTol=0.001  MinStep=1e-09  ToWorkspace=off  RevertToSquareIcSolve=off  NumHomotopyIterations=100  PhasorMode=off  PhasorModeNumHarmonics=1  IndexReductionMethod=DerivativeReplacement  DoDC=off  ResidualTolerance=1e-09  UseLocalSolver=on  LocalSolverChoice=NE_BACKWARD_EULER_ADVANCER  LocalSolverSampleTime=sample_Time  DoFixedCost=on  MaxNonlinIter=3  MaxModeIter=2  ComputeImpulses=off  ImpulseIterations=2  LinearAlgebra=auto  LinearAlgebraNumThread=0  EquationFormulation=NE_TIME_EF  DelaysMemoryBudget=1024  AutomaticFiltering=on  FilteringTimeConstant=0.001  PartitionStorageMethod=AS_NEEDED  PartitionMemoryBudget=1024  PartitionMethod=ROBUST
      settings: SourceProductBaseCode=SS,PW,VE
  World Frame : sm_lib/Frames and Transforms/World Frame
  Wrist_joint : Subsystem
  p : Outport
  pdot : Outport  Port=2
  wires:
  Mux/1 -> p/1
  Mux1/1 -> pdot/1
  [p_1] -> Mux/1
  [pdot_1] -> Mux1/1
  [p_2] -> Mux/2
  [pdot_2] -> Mux1/2
  [p_3] -> Mux/3
  [pdot_3] -> Mux1/3
  [p_4] -> Mux/4
  [pdot_4] -> Mux1/4
  connections:
  RightForeArm/LConn2 -- RightHand/LConn2 -- RightShoulder/LConn2 -- Mechanism Configuration/RConn1 -- World Frame/RConn1 -- RightShoulder_joint/LConn1 -- Solver Configuration1/RConn1
  Elbow_joint/RConn1 -- RightForeArm/LConn1
  RightHand/LConn1 -- Wrist_joint/RConn1
  Wrist_joint/LConn1 -- RightForeArm/RConn1
  RightShoulder/RConn1 -- Elbow_joint/LConn1
  RightShoulder_joint/RConn1 -- RightShoulder/LConn1

== system master_thesis_simulink/Experiments/S2_F0_H2/Experiments/EKF ==
  p_0' : Inport
  v_0' : Inport  Port=2
  markers shoulder : Inport  Port=3
  markers forearm : Inport  Port=4
  markers hand : Inport  Port=5
  Action Port : ActionPort  ActionPortLabel=case [ 2 ]:
  Extended Kalman Filter : MATLAB Function  TreatAsAtomicUnit=on
  Gain1 : Gain  Gain=180/pi
  Scope1 : Scope
  Scope2 : Scope
  Scope4 : Scope
  Terminator : Terminator
  error_FK__EKF : ToWorkspace  VariableName=error_FK__EKF  SaveFormat=Structure With Time  SampleTime=-1
  p_0p - Phi(q_EKF) : MATLAB Function  TreatAsAtomicUnit=on
  p_1 : InportShadow
  p_2 : ToWorkspace  VariableName=p_0p  SaveFormat=Structure With Time  SampleTime=-1
  q_EKF : ToWorkspace  VariableName=q_EKF  SaveFormat=Structure With Time  SampleTime=-1
  v_1 : ToWorkspace  VariableName=v_0p  SaveFormat=Structure With Time  SampleTime=-1
  wires:
  p_0'/1 -> Extended Kalman Filter/1(p_0p), p_2/1
  v_0'/1 -> v_1/1, Extended Kalman Filter/2(v_0p)
  Extended Kalman Filter/1(qk) -> [q_EKF], Gain1/1, Scope4/1
  p_1/1 -> p_0p - Phi(q_EKF)/1(p_0p)
  p_0p - Phi(q_EKF)/1(error_FK) -> error_FK__EKF/1, Scope2/1
  Gain1/1 -> q_EKF/1, Scope1/1  "q_EKF [deg]"
  markers hand/1 -> p_0p - Phi(q_EKF)/5(hand_variables), Extended Kalman Filter/5(hand_variables)
  markers forearm/1 -> p_0p - Phi(q_EKF)/4(forearm_variables), Extended Kalman Filter/4(forearm_variables)
  markers shoulder/1 -> p_0p - Phi(q_EKF)/3(shoulder_variables), Extended Kalman Filter/3(shoulder_variables)
  [q_EKF] -> p_0p - Phi(q_EKF)/2(q_EKF)
  Extended Kalman Filter/2(Pk) -> Terminator/1

== system master_thesis_simulink/Experiments/S2_F0_H2/Experiments/Human arm ==
  note: WRIST-HAND
  note: SHOULDER
  note: ELBOW-FOREARM
  note: B_shoulder
  Elbow_joint : Subsystem
  From3 : From  Commented=on  GotoTag=pShoulder_0  TagVisibility=global
  From4 : From  Commented=on  GotoTag=pForearm_0  TagVisibility=global
  From5 : From  Commented=on  GotoTag=pHand_0  TagVisibility=global
  Goto1 : Goto  Commented=on  GotoTag=pShoulder_i_0  TagVisibility=global
  Goto2 : Goto  Commented=on  GotoTag=pForearm_i_0  TagVisibility=global
  Goto3 : Goto  Commented=on  GotoTag=pHand_i_0  TagVisibility=global
  MATLAB Function2 : MATLAB Function  Commented=on  TreatAsAtomicUnit=on
  MATLAB Function3 : MATLAB Function  Commented=on  TreatAsAtomicUnit=on
  MATLAB Function4 : MATLAB Function  Commented=on  TreatAsAtomicUnit=on
  Markers : Subsystem  Commented=on
  Mechanism Configuration : sm_lib/Utilities/Mechanism Configuration  UniformGravity=Constant  GravityVector=[0 0 -9.80665]  GravityUnits=m/s^2  LinearizationDelta=0.001  JointModeTransitionNonlinearIterations=2
  Mux : Mux  Inputs=m
  Mux1 : Mux  Inputs=m
  RightForeArm : Subsystem
  RightHand : Subsystem
  RightShoulder : Subsystem
  RightShoulder_joint : Subsystem
  Solver Configuration1 : nesl_utility/Solver Configuration  PhysicalDomain=network_engine_domain  SubClassName=solver  LeftPortType=input  RightPortType=generic  Tones=[]  Harmonics=[]  SimulateNoise=off  Profile=off  UseLocalSampling=off  EnableSwitchedLinearOptims=on  FrequencyDomain=off  UseCCode=off  RelTol=0.001  AbsTol=0.001  MinStep=1e-09  ToWorkspace=off  RevertToSquareIcSolve=off  NumHomotopyIterations=100  PhasorMode=off  PhasorModeNumHarmonics=1  IndexReductionMethod=DerivativeReplacement  DoDC=off  ResidualTolerance=1e-09  UseLocalSolver=off  LocalSolverChoice=NE_BACKWARD_EULER_ADVANCER  LocalSolverSampleTime=0.001  DoFixedCost=off  MaxNonlinIter=3  MaxModeIter=2  ComputeImpulses=off  ImpulseIterations=2  LinearAlgebra=auto  LinearAlgebraNumThread=0  EquationFormulation=NE_TIME_EF  DelaysMemoryBudget=1024  AutomaticFiltering=on  FilteringTimeConstant=0.001  PartitionStorageMethod=AS_NEEDED  PartitionMemoryBudget=1024  PartitionMethod=ROBUST
      settings: SourceProductBaseCode=SS,PW,VE
  World Frame : sm_lib/Frames and Transforms/World Frame
  Wrist_joint : Subsystem
  p : Outport
  pdot : Outport  Port=2
  wires:
  MATLAB Function4/1(y) -> Goto3/1
  From5/1 -> MATLAB Function4/1(hand)
  From4/1 -> MATLAB Function3/1(forearm)
  MATLAB Function3/1(y) -> Goto2/1
  MATLAB Function2/1(y) -> Goto1/1
  From3/1 -> MATLAB Function2/1(shoulder)
  Mux1/1 -> pdot/1
  Mux/1 -> p/1
  connections:
  RightShoulder_joint/RConn1 -- RightShoulder/LConn1
  RightShoulder/RConn1 -- Elbow_joint/LConn1
  Wrist_joint/LConn1 -- RightForeArm/RConn1
  RightHand/LConn1 -- Wrist_joint/RConn1
  Elbow_joint/RConn1 -- RightForeArm/LConn1
  World Frame/RConn1 -- Solver Configuration1/RConn1 -- RightShoulder/LConn2 -- RightHand/LConn2 -- RightForeArm/LConn2 -- RightShoulder_joint/LConn1 -- Mechanism Configuration/RConn1

== system master_thesis_simulink/Experiments/S2_F0_H2/Experiments/Human arm_exp ==
  note: WRIST-HAND
  note: ELBOW-FOREARM
  note: SHOULDER
  note: B_shoulder
  Elbow_joint : Subsystem
  Markers : Subsystem  Commented=on
  Mechanism Configuration : sm_lib/Utilities/Mechanism Configuration  UniformGravity=Constant  GravityVector=[0 0 -9.80665]  GravityUnits=m/s^2  LinearizationDelta=0.001  JointModeTransitionNonlinearIterations=2
  Mux : Mux  Inputs=m
  Mux1 : Mux  Inputs=m
  RightForeArm : Subsystem
  RightHand : Subsystem
  RightShoulder : Subsystem
  RightShoulder_joint : Subsystem
  Solver Configuration1 : nesl_utility/Solver Configuration  PhysicalDomain=network_engine_domain  SubClassName=solver  LeftPortType=input  RightPortType=generic  Tones=[]  Harmonics=[]  SimulateNoise=off  Profile=off  UseLocalSampling=off  EnableSwitchedLinearOptims=on  FrequencyDomain=off  UseCCode=off  RelTol=0.001  AbsTol=0.001  MinStep=1e-09  ToWorkspace=off  RevertToSquareIcSolve=off  NumHomotopyIterations=100  PhasorMode=off  PhasorModeNumHarmonics=1  IndexReductionMethod=DerivativeReplacement  DoDC=off  ResidualTolerance=1e-09  UseLocalSolver=off  LocalSolverChoice=NE_BACKWARD_EULER_ADVANCER  LocalSolverSampleTime=0.001  DoFixedCost=off  MaxNonlinIter=3  MaxModeIter=2  ComputeImpulses=off  ImpulseIterations=2  LinearAlgebra=auto  LinearAlgebraNumThread=0  EquationFormulation=NE_TIME_EF  DelaysMemoryBudget=1024  AutomaticFiltering=on  FilteringTimeConstant=0.001  PartitionStorageMethod=AS_NEEDED  PartitionMemoryBudget=1024  PartitionMethod=ROBUST
      settings: SourceProductBaseCode=SS,PW,VE
  World Frame : sm_lib/Frames and Transforms/World Frame
  Wrist_joint : Subsystem
  p : Outport
  pdot : Outport  Port=2
  wires:
  Mux1/1 -> pdot/1
  Mux/1 -> p/1
  connections:
  Elbow_joint/RConn1 -- RightForeArm/LConn1
  RightShoulder_joint/LConn1 -- World Frame/RConn1 -- Mechanism Configuration/RConn1 -- Solver Configuration1/RConn1 -- RightShoulder/LConn2 -- RightHand/LConn2 -- RightForeArm/LConn2
  Wrist_joint/LConn1 -- RightForeArm/RConn1
  Elbow_joint/LConn1 -- RightShoulder/RConn1
  RightHand/LConn1 -- Wrist_joint/RConn1
  RightShoulder/LConn1 -- RightShoulder_joint/RConn1
